simulink model "Suspension_System_Analysis_Sim"  (R2017b)
settings: Solver=VariableStepAuto  StartTime=0.0  StopTime=50  RelTol=1e-3
settings Model: Creator=Oguzhan  LastModifiedBy=Oguzhan

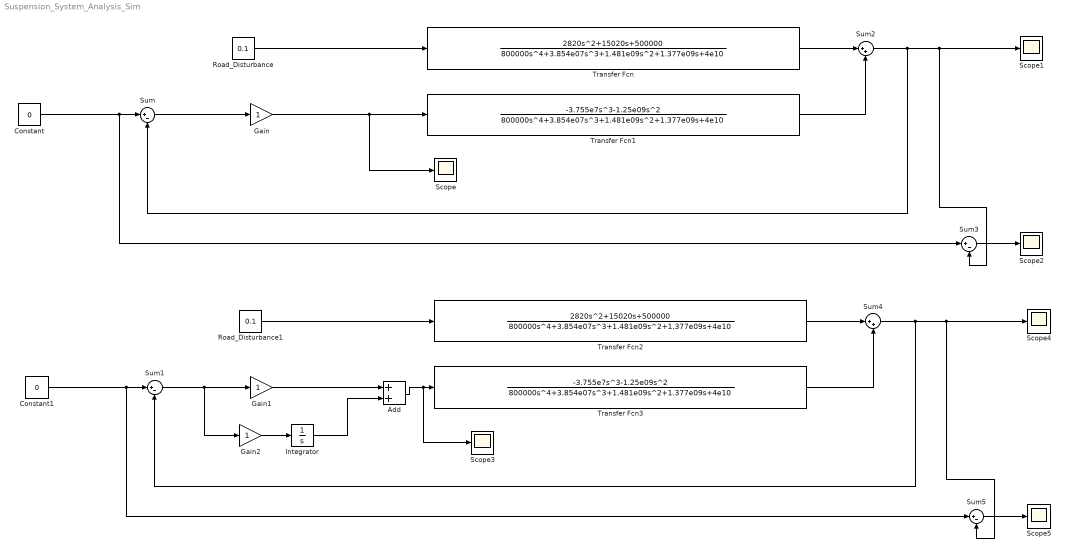
== system Suspension_System_Analysis_Sim ==
  Add : Sum
  Constant : Constant  Value=0
  Constant1 : Constant  Value=0
  Gain : Gain
  Gain1 : Gain
  Gain2 : Gain
  Integrator : Integrator
  Road_Disturbance : Constant  Value=0.1
  Road_Disturbance1 : Constant  Value=0.1
  Scope{,1..5} (6 alike) : Scope
  Sum{,1,3,5} (4 alike) : Sum  Inputs=|+-
  Sum2 : Sum  Inputs=|++
  Sum4 : Sum  Inputs=|++
  Transfer Fcn : TransferFcn  Numerator=[2820 15020 500000]  Denominator=[800000 3.854e07 1.481e09 1.377e09 4e10]
  Transfer Fcn1 : TransferFcn  Numerator=[-3.755e7 -1.25e09 0 0]  Denominator=[800000 3.854e07 1.481e09 1.377e09 4e10]
  Transfer Fcn2 : TransferFcn  Numerator=[2820 15020 500000]  Denominator=[800000 3.854e07 1.481e09 1.377e09 4e10]
  Transfer Fcn3 : TransferFcn  Numerator=[-3.755e7 -1.25e09 0 0]  Denominator=[800000 3.854e07 1.481e09 1.377e09 4e10]
  wires:
  Constant/1 -> Sum3/1, Sum/1
  Gain/1 -> Transfer Fcn1/1, Scope/1
  Road_Disturbance/1 -> Transfer Fcn/1
  Transfer Fcn/1 -> Sum2/1
  Transfer Fcn1/1 -> Sum2/2
  Sum2/1 -> Sum3/2, Scope1/1, Sum/2
  Sum3/1 -> Scope2/1
  Sum/1 -> Gain/1
  Sum5/1 -> Scope5/1
  Transfer Fcn2/1 -> Sum4/1
  Road_Disturbance1/1 -> Transfer Fcn2/1
  Constant1/1 -> Sum5/1, Sum1/1
  Sum4/1 -> Sum5/2, Scope4/1, Sum1/2
  Sum1/1 -> Gain2/1, Gain1/1
  Transfer Fcn3/1 -> Sum4/2
  Gain1/1 -> Add/1
  Add/1 -> Scope3/1, Transfer Fcn3/1
  Gain2/1 -> Integrator/1
  Integrator/1 -> Add/2
